simulink model "PidNvidiaCan"  (R2025a)
settings: configuration reference "DeployNVIDIA" (kept outside this file)
undefined symbols (not defined in the file): w_max
libraries: nvidiaCommlib x3, ESys x1
settings Model: DataDictionary=System.sldd  Creator=rodri  LastModifiedBy=mcbti_speedgoat
settings ConfigSetRef: SourceName=DeployNVIDIA

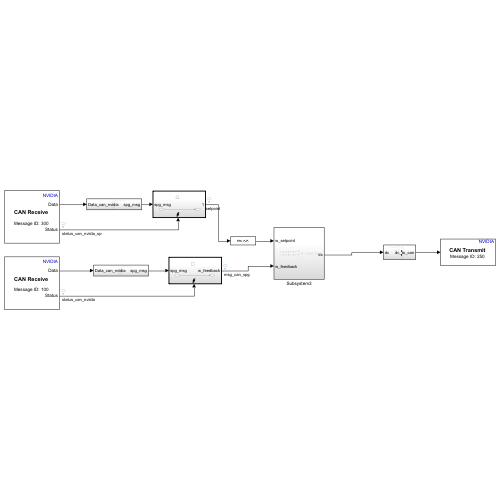
[thumbnail: Simulink's stored preview of the top-level diagram]
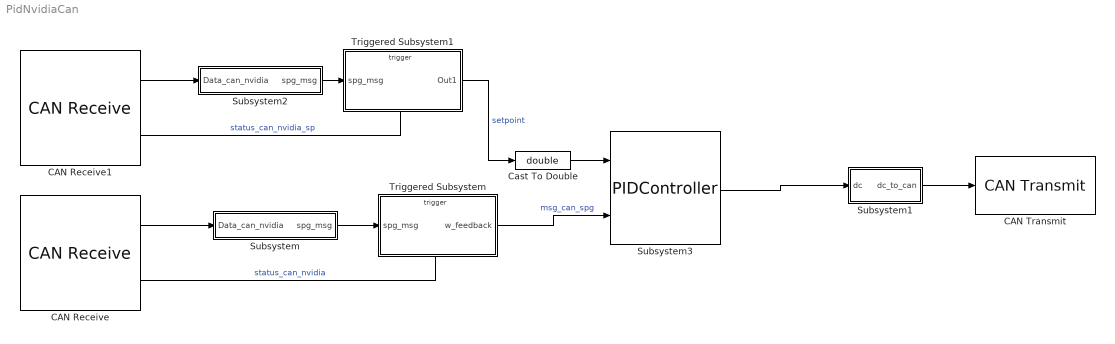
== system PidNvidiaCan ==
  CAN Receive : nvidiaCommlib/CAN Receive  DeviceID=can0  SetupCAN=off  TypeofCAN=Real  OutputDataType=Raw data  IdentifierType=Standard (11-bit identifier)  MessageId=100  MsgLength=8  SampleTime=1e-3  OutputError=off  OutputRemote=off  SimulateUsing=Code generation
  CAN Receive1 : nvidiaCommlib/CAN Receive  DeviceID=can0  SetupCAN=off  TypeofCAN=Real  OutputDataType=Raw data  IdentifierType=Standard (11-bit identifier)  MessageId=300  MsgLength=8  SampleTime=1e-3  OutputError=off  OutputRemote=off  SimulateUsing=Code generation
  CAN Transmit : nvidiaCommlib/CAN Transmit  DeviceID=can0  SetupCAN=off  TypeofCAN=Real  InputDataType=Raw data  BlockingMode_=off  BlockTimeout_=1  OutputStatus=off  IdentifierType=Standard (11-bit identifier)  MessageId=250  MsgLength=8  RemoteFrame=off  SimulateUsing=Code generation
  Cast To Double : DataTypeConversion  OutDataTypeStr=double  SaturateOnIntegerOverflow=off  RndMeth=Floor
  Subsystem : Subsystem
  Subsystem1 : Subsystem
  Subsystem2 : Subsystem
  Subsystem3 : ESys/PIDController  SystemSampleTime=-1  VariantActivationTime=update diagram  EmptyChoice=off  PassThrough=off  PassThroughVariantControl=(default)  EmptyChoiceVariantControl=(default)  AllowFlexibleInterface=on  Latency=0  AutoFrameSizeCalculation=off
  Triggered Subsystem : Subsystem  TreatAsAtomicUnit=on
  Triggered Subsystem1 : Subsystem  TreatAsAtomicUnit=on
  wires:
  CAN Receive/1 -> Subsystem/1(Data_can_nvidia)
  Subsystem/1(spg_msg) -> Triggered Subsystem/1(spg_msg)
  CAN Receive/2 -> Triggered Subsystem/Trigger  "status_can_nvidia"
  Triggered Subsystem1/1(Out1) -> Cast To Double/1  "setpoint"
  Subsystem1/1(dc_to_can) -> CAN Transmit/1
  Cast To Double/1 -> Subsystem3/1
  CAN Receive1/1 -> Subsystem2/1(Data_can_nvidia)
  Subsystem2/1(spg_msg) -> Triggered Subsystem1/1(spg_msg)
  CAN Receive1/2 -> Triggered Subsystem1/Trigger  "status_can_nvidia_sp"
  Triggered Subsystem/1(w_feedback) -> Subsystem3/2  "msg_can_spg"
  Subsystem3/1 -> Subsystem1/1(dc)

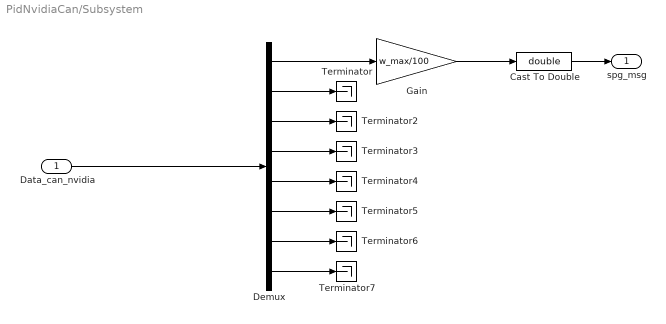
== system PidNvidiaCan/Subsystem ==
  Data_can_nvidia : Inport
  Cast To Double : DataTypeConversion  OutDataTypeStr=double  SaturateOnIntegerOverflow=off  RndMeth=Floor
  Demux : Demux  Outputs=8
  Gain : Gain  Gain=w_max/100
  Terminator{,2..7} (7 alike) : Terminator
  spg_msg : Outport
  wires:
  Data_can_nvidia/1 -> Demux/1
  Demux/8 -> Terminator7/1
  Demux/6 -> Terminator5/1
  Demux/2 -> Terminator/1
  Demux/3 -> Terminator2/1
  Demux/5 -> Terminator4/1
  Demux/4 -> Terminator3/1
  Demux/7 -> Terminator6/1
  Demux/1 -> Gain/1
  Gain/1 -> Cast To Double/1
  Cast To Double/1 -> spg_msg/1

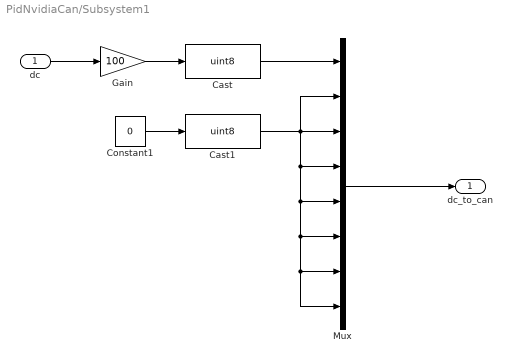
== system PidNvidiaCan/Subsystem1 ==
  dc : Inport
  Cast : DataTypeConversion  OutDataTypeStr=uint8  SaturateOnIntegerOverflow=off  RndMeth=Floor
  Cast1 : DataTypeConversion  OutDataTypeStr=uint8  SaturateOnIntegerOverflow=off  RndMeth=Floor
  Constant1 : Constant  Value=0
  Gain : Gain  Gain=100
  Mux : Mux  Inputs=8
  dc_to_can : Outport
  wires:
  Cast1/1 -> Mux/2, Mux/8, Mux/7, Mux/6, Mux/5, Mux/4, Mux/3
  Cast/1 -> Mux/1
  Constant1/1 -> Cast1/1
  Mux/1 -> dc_to_can/1
  Gain/1 -> Cast/1
  dc/1 -> Gain/1

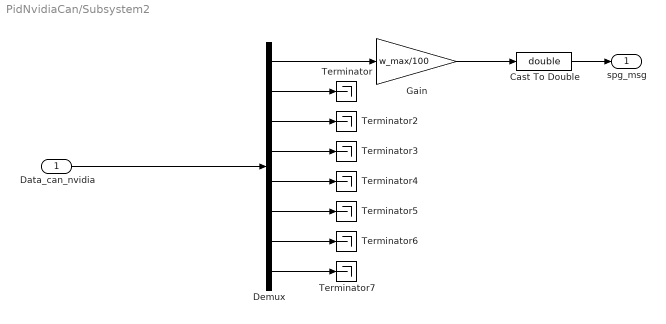
== system PidNvidiaCan/Subsystem2 ==
  Data_can_nvidia : Inport
  Cast To Double : DataTypeConversion  OutDataTypeStr=double  SaturateOnIntegerOverflow=off  RndMeth=Floor
  Demux : Demux  Outputs=8
  Gain : Gain  Gain=w_max/100
  Terminator{,2..7} (7 alike) : Terminator
  spg_msg : Outport
  wires:
  Cast To Double/1 -> spg_msg/1
  Gain/1 -> Cast To Double/1
  Demux/1 -> Gain/1
  Demux/7 -> Terminator6/1
  Demux/4 -> Terminator3/1
  Demux/5 -> Terminator4/1
  Demux/3 -> Terminator2/1
  Demux/2 -> Terminator/1
  Demux/6 -> Terminator5/1
  Demux/8 -> Terminator7/1
  Data_can_nvidia/1 -> Demux/1

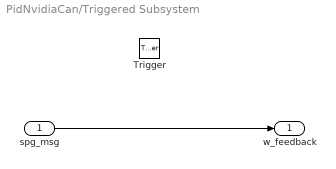
== system PidNvidiaCan/Triggered Subsystem ==
  spg_msg : Inport
  Trigger : TriggerPort  VariantControl=(inherit)
  w_feedback : Outport
  wires:
  spg_msg/1 -> w_feedback/1

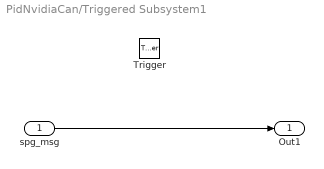
== system PidNvidiaCan/Triggered Subsystem1 ==
  spg_msg : Inport
  Trigger : TriggerPort  VariantControl=(inherit)
  Out1 : Outport
  wires:
  spg_msg/1 -> Out1/1
